simulink model "Adaptive_CT_ur10"  (R2022a)
settings: Solver=ode4  StartTime=0.0  StopTime=15.0  FixedStep=1e-3  RelTol=1e-5
values from neighbouring files (symbols this model uses):
  Kp = 28*diag([14 14 17 10 22 22])    [GuadagniControllore.m]
  Kv = 32*diag([14 14 17 10 22 22])    [GuadagniControllore.m]
undefined symbols (not defined in the file or in its folder): l1, l2, l3, l4, l5, l6, m1, m2, m3, m4, m5, m6, q0, r
libraries: roblocks x3
(part 3 of 9)

== matlab function Adaptive_CT_ur10/CT control/B_matrix ==
  data: param input; B output; q input
function B = B_matrix(param, q)
%#codegen

l1 = param(1);
l2 = param(2);
l3 = param(3);
l4 = param(4);
l5 = param(5);
l6 = param(6);
m1 = param(7);
m2 = param(8);
m3 = param(9);
m4 = param(10);
m5 = param(11);
m6 = param(12);
r = param(13);

q1 = q(1);
q2 = q(2);
q3 = q(3);
q4 = q(4);
q5 = q(5);
q6 = q(6);

%    This function was generated by the Symbolic Math Toolbox version 9.0.
%    06-Jul-2022 11:13:57

t2 = cos(q3);
t3 = cos(q4);
t4 = cos(q5);
t5 = sin(q2);
t6 = sin(q3);
t7 = sin(q4);
t8 = sin(q5);
t9 = q2+q3;
t10 = q2+q5;
t11 = q3+q4;
t12 = l2.^2;
t13 = l3.^2;
t14 = l4.^2;
t15 = l5.^2;
t16 = l6.^2;
t17 = q2.*2.0;
t18 = q3.*2.0;
t19 = q4.*2.0;
t20 = q5.*2.0;
t21 = r.^2;
t31 = -q5;
t22 = cos(t17);
t23 = cos(t20);
t24 = t4.^2;
t25 = l3.*t7;
t26 = q4+t9;
t27 = q5+t9;
t28 = sin(t9);
t29 = sin(t10);
t30 = sin(t11);
t32 = -t20;
t36 = m3.*t13;
t37 = m4.*t13;
t38 = m6.*t13;
t39 = m6.*t15;
t40 = q2+t9;
t42 = l2.*l3.*m3.*t2;
t43 = l2.*l3.*m4.*t2;
t44 = l2.*l3.*m6.*t2;
t45 = l5.*l6.*m6.*t4;
t49 = l2.*l4.*m4.*t5;
t50 = l2.*l4.*m6.*t5;
t52 = q2+t31;
t53 = t9.*2.0;
t54 = t9+t31;
t60 = l2.*l5.*m6.*t2.*t7;
t61 = l2.*l5.*m6.*t3.*t6;
t62 = l3.*l6.*m6.*t3.*t8;
t70 = (m3.*t21)./2.0;
t71 = (m4.*t21)./4.0;
t72 = (m5.*t21)./4.0;
t73 = (m6.*t21)./4.0;
t76 = (m4.*t14)./1.2e+1;
t77 = (m5.*t15)./1.2e+1;
t81 = l2.*l6.*m6.*t2.*t3.*t8;
t82 = l2.*l6.*m6.*t6.*t7.*t8;
t87 = (m6.*t4.*t21)./2.0;
t88 = m6.*t16.*(1.3e+1./1.2e+1);
t33 = cos(t26);
t34 = q5+t26;
t35 = sin(t27);
t41 = cos(t40);
t46 = l5+t25;
t47 = l2.*t30;
t51 = l5.*m6.*t25;
t55 = sin(t52);
t56 = t20+t26;
t58 = l3.*l4.*m4.*t28;
t59 = l3.*l4.*m6.*t28;
t63 = cos(t53);
t64 = -t45;
t65 = t26+t31;
t66 = t26+t32;
t67 = sin(t54);
t68 = -t49;
t69 = -t50;
t75 = t62.*2.0;
t85 = -t62;
t89 = t19+t53;
t91 = (l2.*l6.*m6.*t29)./2.0;
t93 = -t81;
t97 = t24.*t72;
t98 = t24.*t73;
t107 = t24.*t77;
t116 = m5.*t15.*t24.*(-1.0./1.2e+1);
t117 = t24.*t88;
t123 = m6.*t16.*t24.*(-1.3e+1./1.2e+1);
t48 = cos(t34);
t57 = t51.*2.0;
t74 = cos(t56);
t78 = l4.*l5.*m6.*t33;
t79 = cos(t65);
t80 = cos(t66);
t83 = -t58;
t84 = -t59;
t86 = -t75;
t90 = cos(t89);
t92 = l6.*m6.*t4.*t46;
t95 = -t91;
t96 = (l3.*l6.*m6.*t35)./2.0;
t99 = t46+t47;
t103 = t20+t89;
t104 = t33.*t72;
t105 = t33.*t73;
t111 = t32+t89;
t112 = t33.*t77;
t113 = m5.*t21.*t33.*(-1.0./4.0);
t114 = m6.*t21.*t33.*(-1.0./4.0);
t115 = (l2.*l6.*m6.*t55)./2.0;
t119 = (l3.*l6.*m6.*t67)./2.0;
t120 = m5.*t15.*t33.*(-1.0./1.2e+1);
t121 = t33.*t88;
t127 = m6.*t16.*t33.*(-1.3e+1./1.2e+1);
t145 = t39+t51+t71+t72+t73+t76+t77+t85+t88+t97+t98+t116+t123;
t94 = -t79;
t100 = (l4.*l6.*m6.*t48)./2.0;
t101 = (l5.*l6.*m6.*t48)./2.0;
t102 = -t92;
t106 = -t96;
t108 = cos(t103);
t118 = cos(t111);
t122 = -t115;
t124 = -t119;
t125 = (l4.*l6.*m6.*t79)./2.0;
t126 = (l5.*l6.*m6.*t79)./2.0;
t128 = l6.*m6.*t4.*t99;
t129 = (m5.*t15.*t74)./4.8e+1;
t130 = (m5.*t21.*t74)./1.6e+1;
t131 = (m6.*t21.*t74)./1.6e+1;
t133 = (m5.*t15.*t80)./4.8e+1;
t135 = m6.*t16.*t74.*(1.3e+1./4.8e+1);
t136 = (m5.*t21.*t80)./1.6e+1;
t137 = (m6.*t21.*t80)./1.6e+1;
t140 = m6.*t16.*t80.*(1.3e+1./4.8e+1);
t146 = t60+t61+t82+t93+t145;
t148 = t36+t37+t38+t39+t42+t43+t44+t57+t60+t61+t70+t71+t72+t73+t76+t77+t82+t86+t88+t93+t97+t98+t116+t123;
t109 = -t100;
t110 = -t101;
t132 = -t125;
t134 = -t129;
t138 = -t128;
t139 = t48+t94;
t141 = -t135;
t142 = -t136;
t143 = -t137;
t144 = t73.*t139;
t147 = t91+t96+t109+t110+t113+t114+t120+t122+t124+t126+t127+t132;
t149 = t78+t101+t109+t125+t126+t130+t131+t133+t134+t140+t141+t142+t143;
t150 = t83+t84+t106+t124+t149;
t151 = t68+t69+t95+t122+t150;
et1 = t36.*(7.0./1.2e+1)+t37./2.0+t38./2.0+t39./2.0+t42+t43+t44+t51+m2.*t12.*(7.0./1.2e+1)+(m3.*t12)./2.0+(m4.*t12)./2.0+m4.*t14.*(2.5e+1./2.4e+1)+(m6.*t12)./2.0+(m5.*t15)./1.6e+1+m6.*t14+(m1.*t21)./4.0+m6.*t16.*(1.3e+1./1.6e+1)+(m2.*t21)./4.0+(m3.*t21)./4.0+m4.*t21.*(3.0./8.0)+m5.*t21.*(5.0./1.6e+1)+m6.*t21.*(5.0./1.6e+1)+(t36.*t63)./2.0+(t37.*t63)./2.0+(t38.*t63)./2.0-(t39.*t90)./2.0+(l1.^2.*m1)./1.2e+1+l5.*m6.*t47+(m2.*t12.*t22)./2.0+(m3.*t12.*t22)./2.0+(m4.*t12.*t22)./2.0+(m6.*t12.*t22)./2.0+(m5.*t15.*t23)./4.8e+1+m6.*t16.*t23.*(1.3e+1./4.8e+1);
et2 = m5.*t21.*t23.*(-1.0./1.6e+1)-(m6.*t21.*t23)./1.6e+1-(m4.*t14.*t90)./2.4e+1+(m5.*t15.*t90)./4.8e+1+m6.*t16.*t90.*(1.3e+1./4.8e+1)+(m4.*t21.*t90)./8.0-(m5.*t21.*t90)./1.6e+1-(m6.*t21.*t90)./1.6e+1-(m5.*t15.*t108)./9.6e+1-m6.*t16.*t108.*(1.3e+1./9.6e+1)+(m5.*t21.*t108)./3.2e+1+(m6.*t21.*t108)./3.2e+1-(m5.*t15.*t118)./9.6e+1-m6.*t16.*t118.*(1.3e+1./9.6e+1)+(m5.*t21.*t118)./3.2e+1+(m6.*t21.*t118)./3.2e+1+l4.*l6.*m6.*t4.*2.0+l2.*l3.*m3.*t41+l2.*l3.*m4.*t41+l2.*l3.*m6.*t41-(l5.*l6.*m6.*cos(t31+t89))./2.0-(l3.*l6.*m6.*sin(q4+q5))./2.0;
et3 = l2.*l6.*m6.*sin(q5+t11).*(-1.0./2.0)+l2.*l5.*m6.*sin(q2+t26)+(l3.*l6.*m6.*sin(q4+t31))./2.0+l3.*l5.*m6.*sin(t9+t26)-(l2.*l6.*m6.*sin(t10+t26))./2.0+(l2.*l6.*m6.*sin(t11+t31))./2.0-(l3.*l6.*m6.*sin(t26+t27))./2.0+(l2.*l6.*m6.*sin(t26+t52))./2.0+(l3.*l6.*m6.*sin(t26+t54))./2.0+(l5.*l6.*m6.*cos(t9+t19+t27))./2.0;
B = reshape([et1+et2+et3,t151,t150,t149,t147,t144,t151,t36+t37+t38+t39+t42.*2.0+t43.*2.0+t44.*2.0+t57+t60.*2.0+t61.*2.0+t70+t71+t72+t73+t76+t77-t81.*2.0+t82.*2.0+t86+t88+t97+t98+t116+t123+m2.*t12+m3.*t12+m4.*t12+m6.*t12+(m2.*t21)./2.0,t148,t146,t138,t87,t150,t148,t36+t37+t38+t39+t57+t70+t71+t72+t73+t76+t77+t86+t88+t97+t98+t116+t123,t145,t102,t87,t149,t146,t145,t39+t71+t76+(m5.*t15)./2.4e+1+m6.*t16.*(1.3e+1./2.4e+1)+m5.*t21.*(3.0./8.0)+m6.*t21.*(3.0./8.0)-(m5.*t15.*t23)./2.4e+1-m6.*t16.*t23.*(1.3e+1./2.4e+1)+(m5.*t21.*t23)./8.0+(m6.*t21.*t23)./8.0,t64,t87,t147,t138,t102,t64,t72+t73+t77+t88,0.0,t144,t87,t87,t87,0.0,(m6.*t21)./2.0],[6,6]);
